simulink model "pendulum_3d_control_simualtion"  (R2017a)
settings: Solver=FixedStepAuto  StartTime=0.0  StopTime=10  FixedStep=dt  RelTol=1e-3
values from neighbouring files (symbols this model uses):
  dt = 1e-3    (= 0.001)    [f.m]    (also in fJacobian.m; initialize_controller_pendulum3d.m)
  K = lqr(A,B,Q_lqr, R_lqr)    [initialize_controller_pendulum3d.m]
  Ke = KI(:,1:3)    [initialize_controller_pendulum3d.m]
  Ko = KI(:,4:end)    [initialize_controller_pendulum3d.m]
  L = 2.0    (= 2)    [formEKF_pendulum3d.m]    (also in initialize_controller_pendulum3d.m)
  N = inv(C_xyz*inv(B*K - A)*B)    [initialize_controller_pendulum3d.m]
  phi_init = [phix_init, phiy_init]    [initialize_controller_pendulum3d.m]
  pt_init = [x_init, y_init, z_init]    [initialize_controller_pendulum3d.m]
  x_init = 2.619    [initialize_controller_pendulum3d.m]
  y_init = 0    [initialize_controller_pendulum3d.m]
  z_init = 2.24    [initialize_controller_pendulum3d.m]
libraries: sharedTrackingLibrary x3
settings Model: Creator=Jan  LastModifiedBy=Jan

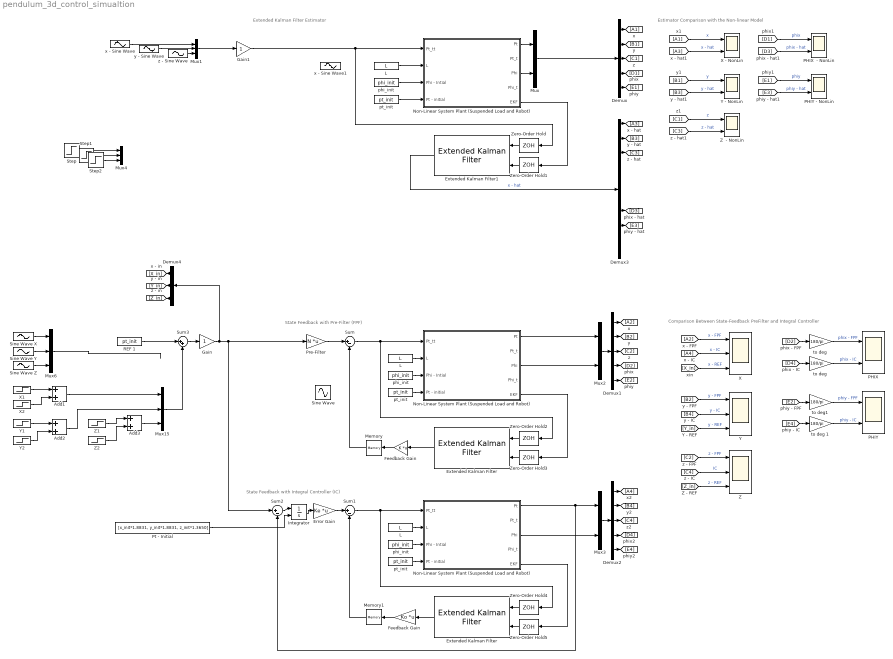
== system pendulum_3d_control_simualtion ==
  note: Extended Kalman Filter Estimator
  note: State Feedback with Pre-Filter (FPF)
  note: Comparison Between State-Feedback PreFilter and Integral Controller
  note: Estimator Comparison with the Non-linear Model
  note: State Feedback with Integral Controller (IC)
  " Error Gain" : Gain  Gain=Ke  Multiplication=Matrix(K*u)
  " Extended Kalman Filter " : sharedTrackingLibrary/Extended Kalman Filter  StateTransitionFcn=f  HasStateTransitionJacobianFcn=on  StateTransitionJacobianFcn=fJacobian  HasAdditiveProcessNoise=Additive  ProcessNoise=Q_EKF  HasTimeVaryingProcessNoise=off  HasStateTransitionFcnExtraArgument=1  InitialState=zeros(10,1)  InitialStateCovariance=P_EKF  MeasurementFcn1=h  HasMeasurementJacobianFcn1=off  MeasurementJacobianFcn1=hJacobian  HasMeasurementEnablePort1=off  HasAdditiveMeasurementNoise1=Additive  MeasurementNoise1=R_EKF  HasTimeVaryingMeasurementNoise1=off  HasMeasurementFcnExtraArgument1=0  MeasurementFcn2=myMeasurementFcn  HasMeasurementJacobianFcn2=off  HasMeasurementEnablePort2=off  HasAdditiveMeasurementNoise2=Additive  MeasurementNoise2=1  HasTimeVaryingMeasurementNoise2=off  HasMeasurementFcnExtraArgument2=0  MeasurementFcn3=myMeasurementFcn  HasMeasurementJacobianFcn3=off  HasMeasurementEnablePort3=off  HasAdditiveMeasurementNoise3=Additive  MeasurementNoise3=1  HasTimeVaryingMeasurementNoise3=off  HasMeasurementFcnExtraArgument3=0  MeasurementFcn4=myMeasurementFcn  HasMeasurementJacobianFcn4=off  HasMeasurementEnablePort4=off  HasAdditiveMeasurementNoise4=Additive  MeasurementNoise4=1  HasTimeVaryingMeasurementNoise4=off  HasMeasurementFcnExtraArgument4=0  MeasurementFcn5=myMeasurementFcn  HasMeasurementJacobianFcn5=off  HasMeasurementEnablePort5=off  HasAdditiveMeasurementNoise5=Additive  MeasurementNoise5=1  HasTimeVaryingMeasurementNoise5=off  HasMeasurementFcnExtraArgument5=0  EnableMultirate=off  StateTransitionFcnSampleTime=1  MeasurementFcn1SampleTime=1  MeasurementFcn2SampleTime=1  MeasurementFcn3SampleTime=1  MeasurementFcn4SampleTime=1  MeasurementFcn5SampleTime=1  UseCurrentEstimator=on  OutputStateCovariance=off  DataType=double  SampleTime=dt  NumberOfMeasurements=1
  " L " : Constant  Value=L
  " Non-Linear System Plant (Suspended Load and Robot) " : Subsystem
  " phi_init " : Constant  Value=phi_init
  " pt_init " : Constant  Value=pt_init
  Add1 : Sum
  Add2 : Sum
  Add3 : Sum
  Demux : Demux  Outputs=5
  Demux1 : Demux  Outputs=5
  Demux2 : Demux  Outputs=5
  Demux3 : Demux  Outputs=10
  Demux4 : Demux  Outputs=3
  "Extended Kalman Filter " : sharedTrackingLibrary/Extended Kalman Filter  StateTransitionFcn=f  HasStateTransitionJacobianFcn=on  StateTransitionJacobianFcn=fJacobian  HasAdditiveProcessNoise=Additive  ProcessNoise=Q_EKF  HasTimeVaryingProcessNoise=off  HasStateTransitionFcnExtraArgument=1  InitialState=zeros(10,1)  InitialStateCovariance=P_EKF  MeasurementFcn1=h  HasMeasurementJacobianFcn1=off  MeasurementJacobianFcn1=hJacobian  HasMeasurementEnablePort1=off  HasAdditiveMeasurementNoise1=Additive  MeasurementNoise1=R_EKF  HasTimeVaryingMeasurementNoise1=off  HasMeasurementFcnExtraArgument1=0  MeasurementFcn2=myMeasurementFcn  HasMeasurementJacobianFcn2=off  HasMeasurementEnablePort2=off  HasAdditiveMeasurementNoise2=Additive  MeasurementNoise2=1  HasTimeVaryingMeasurementNoise2=off  HasMeasurementFcnExtraArgument2=0  MeasurementFcn3=myMeasurementFcn  HasMeasurementJacobianFcn3=off  HasMeasurementEnablePort3=off  HasAdditiveMeasurementNoise3=Additive  MeasurementNoise3=1  HasTimeVaryingMeasurementNoise3=off  HasMeasurementFcnExtraArgument3=0  MeasurementFcn4=myMeasurementFcn  HasMeasurementJacobianFcn4=off  HasMeasurementEnablePort4=off  HasAdditiveMeasurementNoise4=Additive  MeasurementNoise4=1  HasTimeVaryingMeasurementNoise4=off  HasMeasurementFcnExtraArgument4=0  MeasurementFcn5=myMeasurementFcn  HasMeasurementJacobianFcn5=off  HasMeasurementEnablePort5=off  HasAdditiveMeasurementNoise5=Additive  MeasurementNoise5=1  HasTimeVaryingMeasurementNoise5=off  HasMeasurementFcnExtraArgument5=0  EnableMultirate=off  StateTransitionFcnSampleTime=1  MeasurementFcn1SampleTime=1  MeasurementFcn2SampleTime=1  MeasurementFcn3SampleTime=1  MeasurementFcn4SampleTime=1  MeasurementFcn5SampleTime=1  UseCurrentEstimator=on  OutputStateCovariance=off  DataType=double  SampleTime=dt  NumberOfMeasurements=1
  Extended Kalman Filter1 : sharedTrackingLibrary/Extended Kalman Filter  StateTransitionFcn=f  HasStateTransitionJacobianFcn=on  StateTransitionJacobianFcn=fJacobian  HasAdditiveProcessNoise=Additive  ProcessNoise=Q_EKF  HasTimeVaryingProcessNoise=off  HasStateTransitionFcnExtraArgument=1  InitialState=zeros(10,1)  InitialStateCovariance=P_EKF  MeasurementFcn1=h  HasMeasurementJacobianFcn1=off  MeasurementJacobianFcn1=hJacobian  HasMeasurementEnablePort1=off  HasAdditiveMeasurementNoise1=Additive  MeasurementNoise1=R_EKF  HasTimeVaryingMeasurementNoise1=off  HasMeasurementFcnExtraArgument1=0  MeasurementFcn2=myMeasurementFcn  HasMeasurementJacobianFcn2=off  HasMeasurementEnablePort2=off  HasAdditiveMeasurementNoise2=Additive  MeasurementNoise2=1  HasTimeVaryingMeasurementNoise2=off  HasMeasurementFcnExtraArgument2=0  MeasurementFcn3=myMeasurementFcn  HasMeasurementJacobianFcn3=off  HasMeasurementEnablePort3=off  HasAdditiveMeasurementNoise3=Additive  MeasurementNoise3=1  HasTimeVaryingMeasurementNoise3=off  HasMeasurementFcnExtraArgument3=0  MeasurementFcn4=myMeasurementFcn  HasMeasurementJacobianFcn4=off  HasMeasurementEnablePort4=off  HasAdditiveMeasurementNoise4=Additive  MeasurementNoise4=1  HasTimeVaryingMeasurementNoise4=off  HasMeasurementFcnExtraArgument4=0  MeasurementFcn5=myMeasurementFcn  HasMeasurementJacobianFcn5=off  HasMeasurementEnablePort5=off  HasAdditiveMeasurementNoise5=Additive  MeasurementNoise5=1  HasTimeVaryingMeasurementNoise5=off  HasMeasurementFcnExtraArgument5=0  EnableMultirate=off  StateTransitionFcnSampleTime=1  MeasurementFcn1SampleTime=1  MeasurementFcn2SampleTime=1  MeasurementFcn3SampleTime=1  MeasurementFcn4SampleTime=1  MeasurementFcn5SampleTime=1  UseCurrentEstimator=on  OutputStateCovariance=off  DataType=double  SampleTime=dt  NumberOfMeasurements=1
  Feedback Gain : Gain  Gain=K  Multiplication=Matrix(K*u)
  "Feedback Gain " : Gain  Gain=Ko  Multiplication=Matrix(K*u)
  Gain : Gain
  Gain1 : Gain
  Integrator : Integrator  InitialConditionSource=external
  L : Constant  Value=L
  "L " : Constant  Value=L
  Memory : Memory
  Memory1 : Memory
  Mux : Mux  Inputs=2
  Mux{1,4,6,15} (4 alike) : Mux  Inputs=3
  Mux2 : Mux  Inputs=2
  Mux3 : Mux  Inputs=2
  Non-Linear System Plant (Suspended Load and Robot) : Subsystem
  "Non-Linear System Plant (Suspended Load and Robot) " : Subsystem
  "PHIX " : Scope  NumInputPorts=2
  PHIX  - NonLin : Scope  NumInputPorts=2
  "PHIY " : Scope  NumInputPorts=2
  PHIY - NonLin : Scope  NumInputPorts=2
  Pre-Filter : Gain  Gain=N  Multiplication=Matrix(K*u)
  Pt - Initial : Constant  Value=[x_init*1.8831, y_init*1.8831, z_init*1.3650]
  REF 1 : Constant  Value=pt_init
  Sine Wave : Sin  Amplitude=0.75  Bias=2.0  Frequency=2*pi*0.05  SampleTime=0
  Sine Wave X : Sin  Amplitude=0.5  Frequency=2*pi*0.07  SampleTime=0
  Sine Wave Y : Sin  Amplitude=0.3  Frequency=2*pi*0.09  SampleTime=0
  Sine Wave Z : Sin  Amplitude=0.25  Frequency=2*pi*0.15  SampleTime=0
  Step : Step  Time=0  SampleTime=0
  Step1 : Step  Time=0  SampleTime=0
  Step2 : Step  Time=0  SampleTime=0
  Sum : Sum  Inputs=|+-
  Sum1 : Sum  Inputs=|+-
  Sum2 : Sum  Inputs=|+-
  Sum3 : Sum  Inputs=|++
  X : Scope  NumInputPorts=3
  X - NonLin : Scope  NumInputPorts=2
  X1 : Step  After=0.4  SampleTime=0
  X2 : Step  Time=10  After=-0.8  SampleTime=0
  Y : Scope  NumInputPorts=3
  Y - NonLin : Scope  NumInputPorts=2
  Y1 : Step  Time=2  After=0.4  SampleTime=0
  Y2 : Step  Time=13  After=-0.8  SampleTime=0
  Z : Scope  NumInputPorts=3
  Z  - NonLin : Scope  NumInputPorts=2
  Z1 : Step  Time=3  After=0.4  SampleTime=0
  Z2 : Step  Time=9  After=-0.2  SampleTime=0
  Zero-Order Hold{,1..5} (6 alike) : ZeroOrderHold  SampleTime=dt
  phi_init : Constant  Value=phi_init
  "phi_init " : Constant  Value=phi_init
  "pt_init " : Constant  Value=pt_init
  "pt_init " : Constant  Value=pt_init
  to deg : Gain  Gain=180/pi
  "to deg " : Gain  Gain=180/pi
  to deg 1 : Gain  Gain=180/pi
  to deg1 : Gain  Gain=180/pi
  x - Sine Wave : Sin  Frequency=2*pi*0.5  Phase=pi/2  SampleTime=0
  x - Sine Wave1 : Sin  Amplitude=0.75  Bias=2  Frequency=2*pi*0.05  SampleTime=0
  y - Sine Wave : Sin  Frequency=2*pi*0.8  SampleTime=0
  z - Sine Wave : Sin  Amplitude=2  Frequency=2*pi*1  SampleTime=0
  wires:
  phi_init/1 -> Non-Linear System Plant (Suspended Load and Robot)/3(Phi - Intial)
  "pt_init "/1 -> Non-Linear System Plant (Suspended Load and Robot)/4(Pt - initial)
  Zero-Order Hold1/1 -> Extended Kalman Filter1/2
  Zero-Order Hold/1 -> Extended Kalman Filter1/1
  Extended Kalman Filter1/1 -> Demux3/1  "x - hat"
  Demux3/1 -> [A3]
  Demux3/2 -> [B3]
  Demux3/3 -> [C3]
  Demux3/8 -> [E3]
  Demux3/7 -> [D3]
  Non-Linear System Plant (Suspended Load and Robot)/1(Pt) -> Mux/1
  [C1] -> Z  - NonLin/1  "z"
  [B1] -> Y - NonLin/1  "y"
  [E1] -> PHIY - NonLin/1  "phiy"
  [D3] -> PHIX  - NonLin/2  "phix - hat"
  [A3] -> X - NonLin/2  "x - hat"
  [D1] -> PHIX  - NonLin/1  "phix"
  [A1] -> X - NonLin/1  "x"
  [E3] -> PHIY - NonLin/2  "phiy - hat"
  [B3] -> Y - NonLin/2  "y - hat"
  [C3] -> Z  - NonLin/2  "z - hat"
  x - Sine Wave/1 -> Mux1/1
  y - Sine Wave/1 -> Mux1/2
  z - Sine Wave/1 -> Mux1/3
  Mux/1 -> Demux/1
  Non-Linear System Plant (Suspended Load and Robot)/5(EKF) -> Zero-Order Hold1/1
  Non-Linear System Plant (Suspended Load and Robot)/3(Phi) -> Mux/2
  Demux/1 -> [A1]
  Demux/2 -> [B1]
  Demux/3 -> [C1]
  Demux/4 -> [D1]
  Demux/5 -> [E1]
  L/1 -> Non-Linear System Plant (Suspended Load and Robot)/2(L)
  "L "/1 -> "Non-Linear System Plant (Suspended Load and Robot) "/2(L)
  "Non-Linear System Plant (Suspended Load and Robot) "/3(Phi) -> Mux2/2
  "Non-Linear System Plant (Suspended Load and Robot) "/5(EKF) -> Zero-Order Hold3/1
  "Non-Linear System Plant (Suspended Load and Robot) "/1(Pt) -> Mux2/1
  "Extended Kalman Filter "/1 -> Feedback Gain/1
  Zero-Order Hold2/1 -> "Extended Kalman Filter "/1
  Zero-Order Hold3/1 -> "Extended Kalman Filter "/2
  Sum/1 -> "Non-Linear System Plant (Suspended Load and Robot) "/1(Pt_tt), Zero-Order Hold2/1
  "pt_init "/1 -> "Non-Linear System Plant (Suspended Load and Robot) "/4(Pt - initial)
  "phi_init "/1 -> "Non-Linear System Plant (Suspended Load and Robot) "/3(Phi - Intial)
  Mux2/1 -> Demux1/1
  Demux1/4 -> [D2]
  Demux1/3 -> [C2]
  Demux1/1 -> [A2]
  Demux1/2 -> [B2]
  Demux1/5 -> [E2]
  Feedback Gain/1 -> Memory/1
  Memory/1 -> Sum/2
  Pre-Filter/1 -> Sum/1
  [A2] -> X/1  "x - FPF"
  [X_in] -> X/3  "x - REF"
  [A4] -> X/2  "x - IC"
  [B2] -> Y/1  "y - FPF"
  [Z_in] -> Z/3  "z - REF"
  [C2] -> Z/1  "z - FPF"
  [Y_in] -> Y/3  "y - REF"
  to deg/1 -> "PHIX "/1  "phix - FPF"
  "to deg "/1 -> "PHIX "/2  "phix - IC"
  to deg 1/1 -> "PHIY "/2  "phiy - IC"
  to deg1/1 -> "PHIY "/1  "phiy - FPF"
  [D2] -> to deg/1
  [E2] -> to deg1/1
  Sum2/1 -> Integrator/1
  " Error Gain"/1 -> Sum1/1
  Memory1/1 -> Sum1/2
  "Feedback Gain "/1 -> Memory1/1
  " phi_init "/1 -> " Non-Linear System Plant (Suspended Load and Robot) "/3(Phi - Intial)
  " pt_init "/1 -> " Non-Linear System Plant (Suspended Load and Robot) "/4(Pt - initial)
  Sum1/1 -> Zero-Order Hold4/1, " Non-Linear System Plant (Suspended Load and Robot) "/1(Pt_tt)
  Zero-Order Hold5/1 -> " Extended Kalman Filter "/2
  Zero-Order Hold4/1 -> " Extended Kalman Filter "/1
  " Extended Kalman Filter "/1 -> "Feedback Gain "/1
  " Non-Linear System Plant (Suspended Load and Robot) "/1(Pt) -> Mux3/1, Sum2/2
  " Non-Linear System Plant (Suspended Load and Robot) "/5(EKF) -> Zero-Order Hold5/1
  " L "/1 -> " Non-Linear System Plant (Suspended Load and Robot) "/2(L)
  Demux2/4 -> [D4]
  Demux2/5 -> [E4]
  Mux3/1 -> Demux2/1
  Demux2/1 -> [A4]
  Demux2/2 -> [B4]
  Demux2/3 -> [C4]
  [B4] -> Y/2  "y - IC"
  [C4] -> Z/2  "IC"
  [D4] -> "to deg "/1
  [E4] -> to deg 1/1
  " Non-Linear System Plant (Suspended Load and Robot) "/3(Phi) -> Mux3/2
  Integrator/1 -> " Error Gain"/1
  Demux4/1 -> [X_in]
  Demux4/2 -> [Y_in]
  Demux4/3 -> [Z_in]
  Gain/1 -> Demux4/1, Sum2/1, Pre-Filter/1
  Gain1/1 -> Zero-Order Hold/1, Non-Linear System Plant (Suspended Load and Robot)/1(Pt_tt)
  Y2/1 -> Add2/2
  Z1/1 -> Add3/1
  X2/1 -> Add1/2
  Y1/1 -> Add2/1
  Add2/1 -> Mux15/2
  Add3/1 -> Mux15/3
  X1/1 -> Add1/1
  Z2/1 -> Add3/2
  Add1/1 -> Mux15/1
  Sine Wave Y/1 -> Mux6/2
  Sine Wave Z/1 -> Mux6/3
  Sine Wave X/1 -> Mux6/1
  Pt - Initial/1 -> Integrator/2
  Sum3/1 -> Gain/1
  Mux15/1 -> Sum3/2
  Mux1/1 -> Gain1/1
  Step/1 -> Mux4/1
  Step1/1 -> Mux4/2
  Step2/1 -> Mux4/3
  REF 1/1 -> Sum3/1
  Mux6/1 -> ?

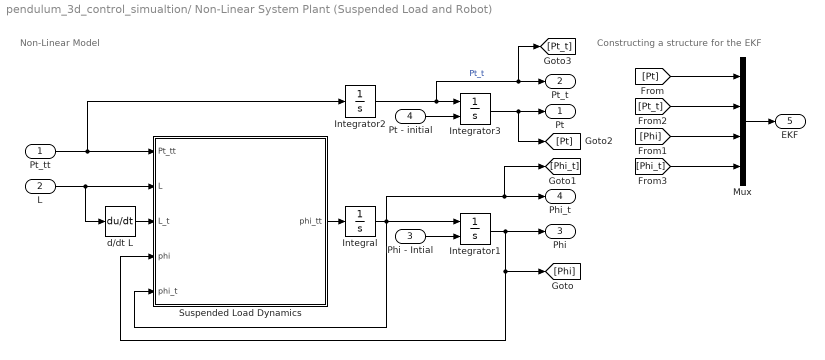
== system pendulum_3d_control_simualtion/ Non-Linear System Plant (Suspended Load and Robot)  ==
  note: Non-Linear Model
  note: Constructing a structure for the EKF
  Pt_tt : Inport
  L : Inport  Port=2
  Phi - Intial : Inport  Port=3
  Pt - initial : Inport  Port=4
  Integral : Integrator  InitialCondition=[0 0]
  Integrator1 : Integrator  InitialConditionSource=external
  Integrator2 : Integrator  InitialCondition=[0 0 0]
  Integrator3 : Integrator  InitialConditionSource=external
  Mux : Mux
  Suspended Load Dynamics : MATLAB Function  TreatAsAtomicUnit=on
  d/dt L : Derivative
  Pt : Outport
  Pt_t : Outport  Port=2
  Phi : Outport  Port=3
  Phi_t : Outport  Port=4
  EKF : Outport  Port=5
  wires:
  Pt_tt/1 -> Integrator2/1, Suspended Load Dynamics/1(Pt_tt)
  Integrator3/1 -> [Pt], Pt/1
  Suspended Load Dynamics/1(phi_tt) -> Integral/1
  Integrator2/1 -> [Pt_t], Pt_t/1, Integrator3/1  "Pt_t"
  Pt - initial/1 -> Integrator3/2
  L/1 -> d/dt L/1, Suspended Load Dynamics/2(L)
  d/dt L/1 -> Suspended Load Dynamics/3(L_t)
  Integrator1/1 -> Phi/1, Suspended Load Dynamics/4(phi), [Phi]
  Phi - Intial/1 -> Integrator1/2
  Integral/1 -> [Phi_t], Phi_t/1, Integrator1/1, Suspended Load Dynamics/5(phi_t)
  Mux/1 -> EKF/1
  [Pt] -> Mux/1
  [Phi] -> Mux/3
  [Phi_t] -> Mux/4
  [Pt_t] -> Mux/2

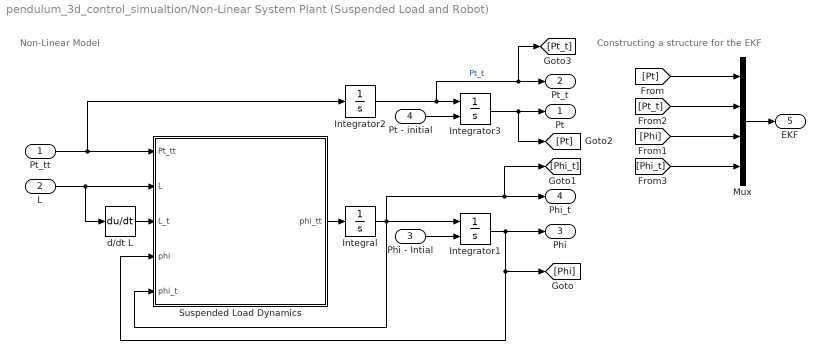
== system pendulum_3d_control_simualtion/Non-Linear System Plant (Suspended Load and Robot) ==
  note: Non-Linear Model
  note: Constructing a structure for the EKF
  Pt_tt : Inport
  L : Inport  Port=2
  Phi - Intial : Inport  Port=3
  Pt - initial : Inport  Port=4
  Integral : Integrator  InitialCondition=[0 0]
  Integrator1 : Integrator  InitialConditionSource=external
  Integrator2 : Integrator  InitialCondition=[0 0 0]
  Integrator3 : Integrator  InitialConditionSource=external
  Mux : Mux
  Suspended Load Dynamics : MATLAB Function  TreatAsAtomicUnit=on
  d/dt L : Derivative
  Pt : Outport
  Pt_t : Outport  Port=2
  Phi : Outport  Port=3
  Phi_t : Outport  Port=4
  EKF : Outport  Port=5
  wires:
  Pt_tt/1 -> Integrator2/1, Suspended Load Dynamics/1(Pt_tt)
  Integrator3/1 -> [Pt], Pt/1
  Suspended Load Dynamics/1(phi_tt) -> Integral/1
  Integrator2/1 -> [Pt_t], Pt_t/1, Integrator3/1  "Pt_t"
  Pt - initial/1 -> Integrator3/2
  L/1 -> d/dt L/1, Suspended Load Dynamics/2(L)
  d/dt L/1 -> Suspended Load Dynamics/3(L_t)
  Integrator1/1 -> Phi/1, Suspended Load Dynamics/4(phi), [Phi]
  Phi - Intial/1 -> Integrator1/2
  Integral/1 -> [Phi_t], Phi_t/1, Integrator1/1, Suspended Load Dynamics/5(phi_t)
  Mux/1 -> EKF/1
  [Pt] -> Mux/1
  [Phi] -> Mux/3
  [Phi_t] -> Mux/4
  [Pt_t] -> Mux/2

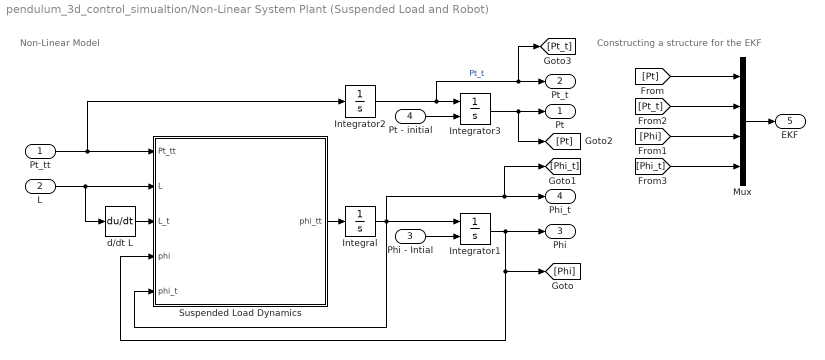
== system pendulum_3d_control_simualtion/Non-Linear System Plant (Suspended Load and Robot)  ==
  note: Constructing a structure for the EKF
  note: Non-Linear Model
  Pt_tt : Inport
  L : Inport  Port=2
  Phi - Intial : Inport  Port=3
  Pt - initial : Inport  Port=4
  Integral : Integrator  InitialCondition=[0 0]
  Integrator1 : Integrator  InitialConditionSource=external
  Integrator2 : Integrator  InitialCondition=[0 0 0]
  Integrator3 : Integrator  InitialConditionSource=external
  Mux : Mux
  Suspended Load Dynamics : MATLAB Function  TreatAsAtomicUnit=on
  d/dt L : Derivative
  Pt : Outport
  Pt_t : Outport  Port=2
  Phi : Outport  Port=3
  Phi_t : Outport  Port=4
  EKF : Outport  Port=5
  wires:
  [Pt_t] -> Mux/2
  [Phi_t] -> Mux/4
  [Phi] -> Mux/3
  [Pt] -> Mux/1
  Mux/1 -> EKF/1
  Integral/1 -> Suspended Load Dynamics/5(phi_t), Integrator1/1, Phi_t/1, [Phi_t]
  Phi - Intial/1 -> Integrator1/2
  Integrator1/1 -> [Phi], Suspended Load Dynamics/4(phi), Phi/1
  d/dt L/1 -> Suspended Load Dynamics/3(L_t)
  L/1 -> Suspended Load Dynamics/2(L), d/dt L/1
  Pt - initial/1 -> Integrator3/2
  Integrator2/1 -> Integrator3/1, Pt_t/1, [Pt_t]  "Pt_t"
  Suspended Load Dynamics/1(phi_tt) -> Integral/1
  Integrator3/1 -> Pt/1, [Pt]
  Pt_tt/1 -> Suspended Load Dynamics/1(Pt_tt), Integrator2/1

== matlab function pendulum_3d_control_simualtion/Non-Linear System Plant (Suspended Load and Robot)/Suspended Load Dynamics ==
  data: Pt_tt input; L input; L_t input; phi_tt output; phi input; phi_t input
function phi_tt = pendulumDynamics(Pt_tt, L, L_t, phi, phi_t)
    % Calculates the dynamics of the suspended load
    % Derives the differential equation for the euler angles
    %
    % Input: 
    %	Pt_tt   : Tool-point acceleration
    %	phi     : Pendulum Angular position euler angles
    %   phit_t  : Pendulum Angular velocity euler angles
    %   L       : Wire length
    %   L_t     : Wire velocity
    %
    %   Output  :
    %   phit_t  : Pendulum Angular acceleration euler angles
    
    % Parameters
    g = 9.81;   % Gravity
    
    % Tool-point acceleration components
    xt_tt = Pt_tt(1); 
    yt_tt = Pt_tt(2); 
    zt_tt = Pt_tt(3);

    % Pendulum euler angles (angular position)
    phix = phi(1);
    phiy = phi(2);

    % Pendulum euler angles (angular velocity)
    phix_t = phi_t(1);
    phiy_t = phi_t(2);
    
     % Pendulum ODE of the euler angles
    % (found from euler-lagrange equation,
    %  derived by the use of Maple)
    phix_tt = (xt_tt*cos(phix) + yt_tt*sin(phix)*sin(phiy) ...
              - zt_tt*sin(phix)*cos(phiy) ...
              - g*sin(phix)*cos(phiy) ...
              - 2*L_t*phix_t ...
              - L*phiy_t^2*sin(phix)*cos(phix)) / L;

    phiy_tt = (- yt_tt*cos(phiy) - zt_tt*sin(phiy) ...
              - g*sin(phiy) + 2*L_t*phiy_t*cos(phix) ...
              + 2*L*phix_t*phiy_t*sin(phix)) ...
              / (L*cos(phix));

    phi_tt = [phix_tt; phiy_tt];

== matlab function pendulum_3d_control_simualtion/Non-Linear System Plant (Suspended Load and Robot) /Suspended Load Dynamics ==
  data: Pt_tt input; L input; L_t input; phi_tt output; phi input; phi_t input
function phi_tt = pendulumDynamics(Pt_tt, L, L_t, phi, phi_t)
    % Calculates the dynamics of the suspended load
    % Derives the differential equation for the euler angles
    %
    % Input: 
    %	Pt_tt   : Tool-point acceleration
    %	phi     : Pendulum Angular position euler angles
    %   phit_t  : Pendulum Angular velocity euler angles
    %   L       : Wire length
    %   L_t     : Wire velocity
    %
    %   Output  :
    %   phit_t  : Pendulum Angular acceleration euler angles
    
    % Parameters
    g = 9.81;   % Gravity
    
    % Tool-point acceleration components
    xt_tt = Pt_tt(1); 
    yt_tt = Pt_tt(2); 
    zt_tt = Pt_tt(3);

    % Pendulum euler angles (angular position)
    phix = phi(1);
    phiy = phi(2);

    % Pendulum euler angles (angular velocity)
    phix_t = phi_t(1);
    phiy_t = phi_t(2);
    
     % Pendulum ODE of the euler angles
    % (found from euler-lagrange equation,
    %  derived by the use of Maple)
    phix_tt = (xt_tt*cos(phix) + yt_tt*sin(phix)*sin(phiy) ...
              - zt_tt*sin(phix)*cos(phiy) ...
              - g*sin(phix)*cos(phiy) ...
              - 2*L_t*phix_t ...
              - L*phiy_t^2*sin(phix)*cos(phix)) / L;

    phiy_tt = (- yt_tt*cos(phiy) - zt_tt*sin(phiy) ...
              - g*sin(phiy) + 2*L_t*phiy_t*cos(phix) ...
              + 2*L*phix_t*phiy_t*sin(phix)) ...
              / (L*cos(phix));

    phi_tt = [phix_tt; phiy_tt];

== matlab function pendulum_3d_control_simualtion/ Non-Linear System Plant (Suspended Load and Robot) /Suspended Load Dynamics ==
  data: Pt_tt input; L input; L_t input; phi_tt output; phi input; phi_t input
function phi_tt = pendulumDynamics(Pt_tt, L, L_t, phi, phi_t)
    % Calculates the dynamics of the suspended load
    % Derives the differential equation for the euler angles
    %
    % Input: 
    %	Pt_tt   : Tool-point acceleration
    %	phi     : Pendulum Angular position euler angles
    %   phit_t  : Pendulum Angular velocity euler angles
    %   L       : Wire length
    %   L_t     : Wire velocity
    %
    %   Output  :
    %   phit_t  : Pendulum Angular acceleration euler angles
    
    % Parameters
    g = 9.81;   % Gravity
    
    % Tool-point acceleration components
    xt_tt = Pt_tt(1); 
    yt_tt = Pt_tt(2); 
    zt_tt = Pt_tt(3);

    % Pendulum euler angles (angular position)
    phix = phi(1);
    phiy = phi(2);

    % Pendulum euler angles (angular velocity)
    phix_t = phi_t(1);
    phiy_t = phi_t(2);
    
     % Pendulum ODE of the euler angles
    % (found from euler-lagrange equation,
    %  derived by the use of Maple)
    phix_tt = (xt_tt*cos(phix) + yt_tt*sin(phix)*sin(phiy) ...
              - zt_tt*sin(phix)*cos(phiy) ...
              - g*sin(phix)*cos(phiy) ...
              - 2*L_t*phix_t ...
              - L*phiy_t^2*sin(phix)*cos(phix)) / L;

    phiy_tt = (- yt_tt*cos(phiy) - zt_tt*sin(phiy) ...
              - g*sin(phiy) + 2*L_t*phiy_t*cos(phix) ...
              + 2*L*phix_t*phiy_t*sin(phix)) ...
              / (L*cos(phix));

    phi_tt = [phix_tt; phiy_tt];
